simulink model "tf_exhaust_cil_temp"  (R2020a)
settings: Solver=FixedStepAuto  StartTime=0.0  StopTime=10.0  RelTol=1e-3
model workspace (MAT data in the model file):
  a0_exhaust_temp = Simulink.Parameter
  a0_exhaust_temp.Value = 0.4
  a0_exhaust_temp.DataType = 'auto'
  a0_exhaust_temp.Dimensions = [1 1]
  b1_exhaust_temp = Simulink.Parameter
  b1_exhaust_temp.Value = 0
  b1_exhaust_temp.DataType = 'auto'
  b1_exhaust_temp.Dimensions = [1 1]
  const_double_to_int = Simulink.Parameter
  const_double_to_int.Value = 100
  const_double_to_int.DataType = 'auto'
  const_double_to_int.Dimensions = [1 1]
  kp_exhaust_temp = Simulink.Parameter
  kp_exhaust_temp.Value = 0.35
  kp_exhaust_temp.DataType = 'auto'
  kp_exhaust_temp.Dimensions = [1 1]
undefined symbols (not defined in the file): ambient_temp, mcp_nominal_rotation
libraries: cstblocks x1
settings Model: Creator=Victor Hugo  LastModifiedBy=ToT_IPMS_03
settings OptimizationCC: ZeroExternalMemoryAtStartup=off  ZeroInternalMemoryAtStartup=off
settings RTWCC: TargetLang=C++
settings GRTTargetCC: TargetLangStandard=C++03 (ISO)  MultiInstanceERTCode=on  CodeInterfacePackaging=C++ class

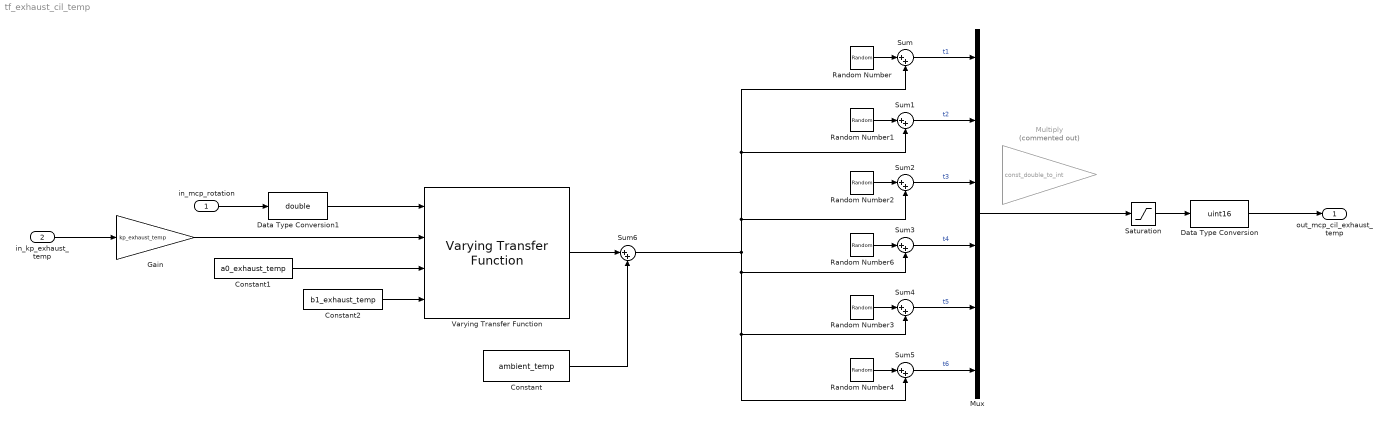
== system tf_exhaust_cil_temp ==
  in_mcp_rotation : Inport  RequirementInfo={} %GIDa_ffd885c5_43d6_4c4b_90af_3fd0d48740d7  OutMin=[0]  OutMax=[mcp_nominal_rotation]  OutDataTypeStr=uint16  Unit=rpm
  in_kp_exhaust_temp : Inport  RequirementInfo={} %GIDa_437868fb_c14d_4c13_8170_33f0b2878206  Port=2  OutMin=[0.008]  OutMax=[0.34]  OutDataTypeStr=double  LockScale=on
  Constant : Constant  Value=ambient_temp
  Constant1 : Constant  RequirementInfo={} %GIDa_ef394db0_9812_4a96_a100_9a20811cda6d  Value=a0_exhaust_temp
  Constant2 : Constant  RequirementInfo={} %GIDa_e66ae3a7_230d_4874_8963_9b28d22fbd3c  Value=b1_exhaust_temp
  Data Type Conversion : DataTypeConversion  RequirementInfo={} %GIDa_90f543ca_322d_4dc7_8d5f_c0d6b9c4964a  OutDataTypeStr=uint16  RndMeth=Nearest  LockScale=on
  Data Type Conversion1 : DataTypeConversion  OutDataTypeStr=double
  Gain : Gain  RequirementInfo={} %GIDa_2083cc78_43ae_4086_ac1f_b5afe6d4d573  Gain=kp_exhaust_temp
  Multiply : Gain  RequirementInfo={} %GIDa_2e84f463_62eb_4e4b_b5a8_7518fe1c4378  Commented=on  Gain=const_double_to_int
  Mux : Mux  RequirementInfo={} %GIDa_ce6722c0_117b_4faa_9a50_850100495796  Inputs=6
  Random Number : RandomNumber  RequirementInfo={} %GIDa_6778de99_1780_4a51_8201_320224b591f9  Variance=2
  Random Number1 : RandomNumber  RequirementInfo={} %GIDa_619e83d6_394d_4ebf_b28b_0b16eb7bebc5  Variance=2  Seed=1
  Random Number2 : RandomNumber  RequirementInfo={} %GIDa_d984c108_e38b_4b36_be1a_c2de570b87e9  Variance=2  Seed=2
  Random Number3 : RandomNumber  RequirementInfo={} %GIDa_c5c6fd81_63f8_4a76_ae2f_8f81b56ce7ea  Mean=1  Variance=2  Seed=6
  Random Number4 : RandomNumber  RequirementInfo={} %GIDa_84d2fcbf_0f2c_4183_a45c_4d89e733cc2f  Variance=2  Seed=5
  Random Number6 : RandomNumber  RequirementInfo={} %GIDa_6a688910_631b_4e08_8077_e80587709949  Variance=2  Seed=3
  Saturation : Saturate  UpperLimit=inf  LowerLimit=0
  Sum : Sum  RequirementInfo={} %GIDa_b8e51aa8_1205_4034_b802_e0e8501a2eaa  Inputs=|++
  Sum1 : Sum  RequirementInfo={} %GIDa_ff06d81a_4b39_4d6a_a1ed_6136227005cb  Inputs=|++
  Sum2 : Sum  RequirementInfo={} %GIDa_ff23c210_d1ae_4a76_9852_33813ab7d599  Inputs=|++
  Sum3 : Sum  RequirementInfo={} %GIDa_c3395440_92c7_4877_a4ca_b2c3a848f3ff  Inputs=|++
  Sum4 : Sum  RequirementInfo={} %GIDa_d824d779_c384_4a32_826f_c2029b83c268  Inputs=|++
  Sum5 : Sum  RequirementInfo={} %GIDa_25973de3_6b98_47c0_a39d_cbd356138551  Inputs=|++
  Sum6 : Sum  Inputs=|++
  Varying Transfer Function : cstblocks/Linear Parameter Varying/Varying Transfer Function  N=1
  out_mcp_cil_exhaust_temp : Outport  RequirementInfo={} %GIDa_3a4f7d42_a5e2_4b83_b11c_6b0c78adfcce  OutMin=[20]  OutMax=[650]  Unit=°C
  wires:
  Sum5/1 -> Mux/6  "t6"
  Data Type Conversion/1 -> out_mcp_cil_exhaust_temp/1
  Constant2/1 -> Varying Transfer Function/4
  Constant1/1 -> Varying Transfer Function/3
  Sum/1 -> Mux/1  "t1"
  Random Number2/1 -> Sum2/1
  Random Number/1 -> Sum/1
  Sum1/1 -> Mux/2  "t2"
  Sum3/1 -> Mux/4  "t4"
  Random Number6/1 -> Sum3/1
  Random Number3/1 -> Sum4/1
  Sum2/1 -> Mux/3  "t3"
  in_mcp_rotation/1 -> Data Type Conversion1/1
  in_kp_exhaust_temp/1 -> Gain/1
  Sum4/1 -> Mux/5  "t5"
  Random Number4/1 -> Sum5/1
  Random Number1/1 -> Sum1/1
  Gain/1 -> Varying Transfer Function/2
  Data Type Conversion1/1 -> Varying Transfer Function/1
  Saturation/1 -> Data Type Conversion/1
  Sum6/1 -> Sum4/2, Sum5/2, Sum3/2, Sum2/2, Sum1/2, Sum/2
  Varying Transfer Function/1 -> Sum6/1
  Constant/1 -> Sum6/2
  Mux/1 -> Saturation/1
